simulink model "schemaSIMULINK"  (R2020b)
settings: Solver=FixedStepAuto  StartTime=0.0  StopTime=35  FixedStep=0.025  RelTol=1e-3
undefined symbols (not defined in the file or in its folder): serial
libraries: instrumentlib x3
settings Model: Creator=eriki  LastModifiedBy=eriki

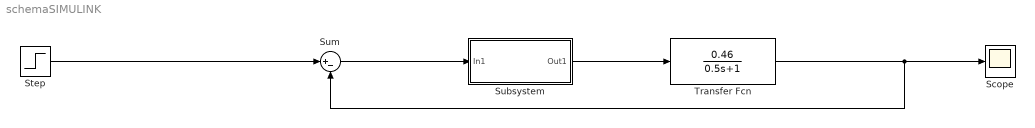
== system schemaSIMULINK ==
  Scope : Scope
  Step : Step  After=120  SampleTime=0.025
  Subsystem : Subsystem
  Sum : Sum  Inputs=|+-
  Transfer Fcn : TransferFcn  Numerator=[0.46]  Denominator=[0.5 1]
  wires:
  Step/1 -> Sum/1
  Sum/1 -> Subsystem/1(In1)
  Subsystem/1(Out1) -> Transfer Fcn/1
  Transfer Fcn/1 -> Scope/1, Sum/2

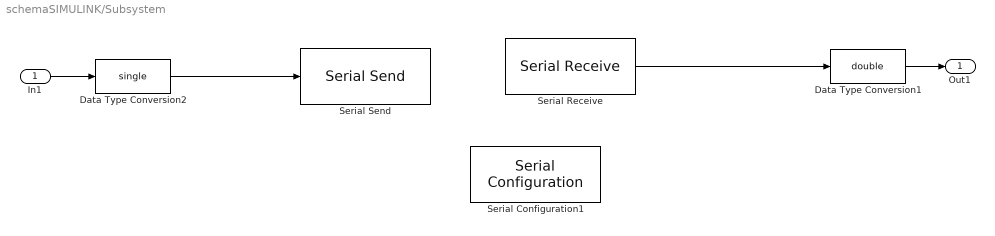
== system schemaSIMULINK/Subsystem ==
  In1 : Inport  SampleTime=0.025
  Data Type Conversion1 : DataTypeConversion  OutDataTypeStr=double
  Data Type Conversion2 : DataTypeConversion  OutDataTypeStr=single
  Serial Configuration1 : instrumentlib/Serial Configuration  Priority=-200000  ComPortMenu=COM11  ComPort=COM11  ObjConstructor=serial('COM11');  BaudRate=9600  DataBits=8  Parity=none  StopBits=1  FlowControl=none  Timeout=10  ByteOrder=LittleEndian
  Serial Receive : instrumentlib/Serial Receive  ComPortMenu=COM11  ComPort=COM11  ObjConstructor=serial('COM11');  Terminator=<none>  DataSize=[1 1]  DataType=uint8  EnableBlockingMode=on  ActionDataUnavailable=Output last received value  CustomValue=0  SampleTime=0.025
  Serial Send : instrumentlib/Serial Send  ComPortMenu=COM11  ComPort=COM11  ObjConstructor=serial('COM11');  Terminator=<none>  EnableBlockingMode=on
  Out1 : Outport  SampleTime=0.025
  wires:
  In1/1 -> Data Type Conversion2/1
  Data Type Conversion1/1 -> Out1/1
  Data Type Conversion2/1 -> Serial Send/1
  Serial Receive/1 -> Data Type Conversion1/1
